simulink model "lab3_sim"  (R2020a)
settings: Solver=VariableStepAuto  StartTime=0.0  StopTime=20  RelTol=1e-3
values from neighbouring files (symbols this model uses):
  d = 0.2    [lab3.m]    (also in lab3_prepp.m = 2)
  h = 1    [lab3.m]    (also in lab3_prepp.m = 3)
  K = 167.61    [lab3.m]
libraries: simulink_extras x4, cstblocks x2
settings Model: Creator=David Wiman  LastModifiedBy=David Wiman

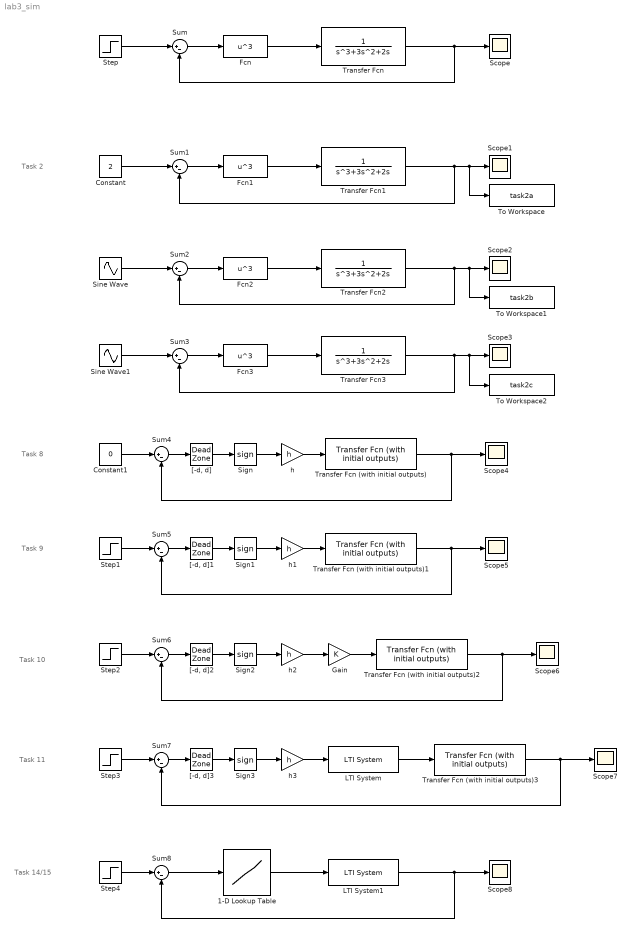
== system lab3_sim ==
  note: Task 11
  note: Task 10
  note: Task 9
  note: Task 8
  note: Task 2
  note: Task 14/15
  1-D Lookup Table : Lookup_n-D  NumberOfTableDimensions=1  BreakpointsForDimension1=[-1 0 1]  Table=[-0.2 0 1]  InternalRulePriority=Speed  RndMeth=Simplest  InputSameDT=on
  Constant : Constant  Value=2
  Constant1 : Constant  Value=0
  Fcn{,1..3} (4 alike) : Fcn  Expr=u^3
  Gain : Gain  Gain=K
  LTI System : cstblocks/LTI System  sys=Flead  IC=[]
  LTI System1 : cstblocks/LTI System  sys=G  IC=[]
  Scope{,1..8} (9 alike) : Scope
  Sign{,1..3} (4 alike) : Signum
  Sine Wave : Sin  Amplitude=0.5  Frequency=100  Phase=pi/2  SampleTime=0
  Sine Wave1 : Sin  Amplitude=0.5  Bias=2  Frequency=100  Phase=pi/2  SampleTime=0
  Step : Step  Time=2  SampleTime=0
  Step1 : Step  Time=5  After=2  SampleTime=0
  Step2 : Step  Time=5  After=2  SampleTime=0
  Step3 : Step  Time=5  After=2  SampleTime=0
  Step4 : Step  Time=0  SampleTime=0
  Sum{,1..8} (9 alike) : Sum  Inputs=|+-
  To Workspace : ToWorkspace  VariableName=task2a  SampleTime=-1
  To Workspace1 : ToWorkspace  VariableName=task2b  SampleTime=-1
  To Workspace2 : ToWorkspace  VariableName=task2c  SampleTime=-1
  Transfer Fcn{,1..3} (4 alike) : TransferFcn  Denominator=[1 3 2 0]
  Transfer Fcn (with initial outputs) : simulink_extras/Additional Linear/Transfer Fcn (with initial outputs)  N=[45]  D=[1 10 9 0]  Y0=0.205  U0=0
  Transfer Fcn (with initial outputs)1 : simulink_extras/Additional Linear/Transfer Fcn (with initial outputs)  N=[45]  D=[1 10 9 0]  Y0=0  U0=0
  Transfer Fcn (with initial outputs)2 : simulink_extras/Additional Linear/Transfer Fcn (with initial outputs)  N=[45]  D=[1 10 9 0]  Y0=0  U0=0
  Transfer Fcn (with initial outputs)3 : simulink_extras/Additional Linear/Transfer Fcn (with initial outputs)  N=[45]  D=[1 10 9 0]  Y0=0  U0=0
  [-d, d]{,1..3} (4 alike) : DeadZone  LowerValue=-d  UpperValue=d  SaturateOnIntegerOverflow=on
  h{,1..3} (4 alike) : Gain  Gain=h
  wires:
  Step/1 -> Sum/1
  Sum/1 -> Fcn/1
  Fcn/1 -> Transfer Fcn/1
  Transfer Fcn/1 -> Sum/2, Scope/1
  Fcn1/1 -> Transfer Fcn1/1
  Sum1/1 -> Fcn1/1
  Constant/1 -> Sum1/1
  Sine Wave/1 -> Sum2/1
  Sum2/1 -> Fcn2/1
  Fcn2/1 -> Transfer Fcn2/1
  Sine Wave1/1 -> Sum3/1
  Sum3/1 -> Fcn3/1
  Fcn3/1 -> Transfer Fcn3/1
  Transfer Fcn1/1 -> Sum1/2, To Workspace/1, Scope1/1
  Transfer Fcn2/1 -> Sum2/2, To Workspace1/1, Scope2/1
  Transfer Fcn3/1 -> Sum3/2, To Workspace2/1, Scope3/1
  Constant1/1 -> Sum4/1
  Transfer Fcn (with initial outputs)/1 -> Sum4/2, Scope4/1
  "[-d, d]"/1 -> Sign/1
  Sign/1 -> h/1
  Sum4/1 -> "[-d, d]"/1
  h/1 -> Transfer Fcn (with initial outputs)/1
  h1/1 -> Transfer Fcn (with initial outputs)1/1
  "[-d, d]1"/1 -> Sign1/1
  Sum5/1 -> "[-d, d]1"/1
  Transfer Fcn (with initial outputs)1/1 -> Sum5/2, Scope5/1
  Sign1/1 -> h1/1
  Step1/1 -> Sum5/1
  "[-d, d]2"/1 -> Sign2/1
  h2/1 -> Gain/1
  Sum6/1 -> "[-d, d]2"/1
  Transfer Fcn (with initial outputs)2/1 -> Sum6/2, Scope6/1
  Step2/1 -> Sum6/1
  Sign2/1 -> h2/1
  Gain/1 -> Transfer Fcn (with initial outputs)2/1
  Transfer Fcn (with initial outputs)3/1 -> Sum7/2, Scope7/1
  Step3/1 -> Sum7/1
  Sum7/1 -> "[-d, d]3"/1
  "[-d, d]3"/1 -> Sign3/1
  Sign3/1 -> h3/1
  h3/1 -> LTI System/1
  LTI System/1 -> Transfer Fcn (with initial outputs)3/1
  1-D Lookup Table/1 -> LTI System1/1
  LTI System1/1 -> Sum8/2, Scope8/1
  Step4/1 -> Sum8/1
  Sum8/1 -> 1-D Lookup Table/1
